simulink model "Progetto_predistorter_2020b"  (R2024b)
settings: Solver=VariableStepAuto  StartTime=0.0  StopTime=30  RelTol=1e-3
libraries: commrflib2 x4, commfilt2 x1
settings Model: Creator=babu9  LastModifiedBy=giorgiomessina
settings SolverCC: AlgebraicLoopSolver=TrustRegion
settings RTWCC: GPUComputeCapability=3.5  DLArmComputeVersion=19.05

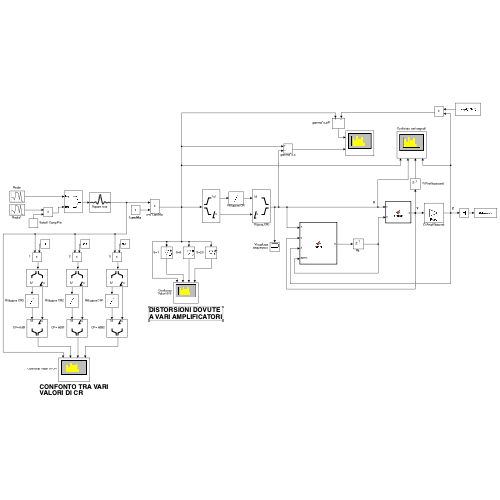
[thumbnail: Simulink's stored preview of the top-level diagram]
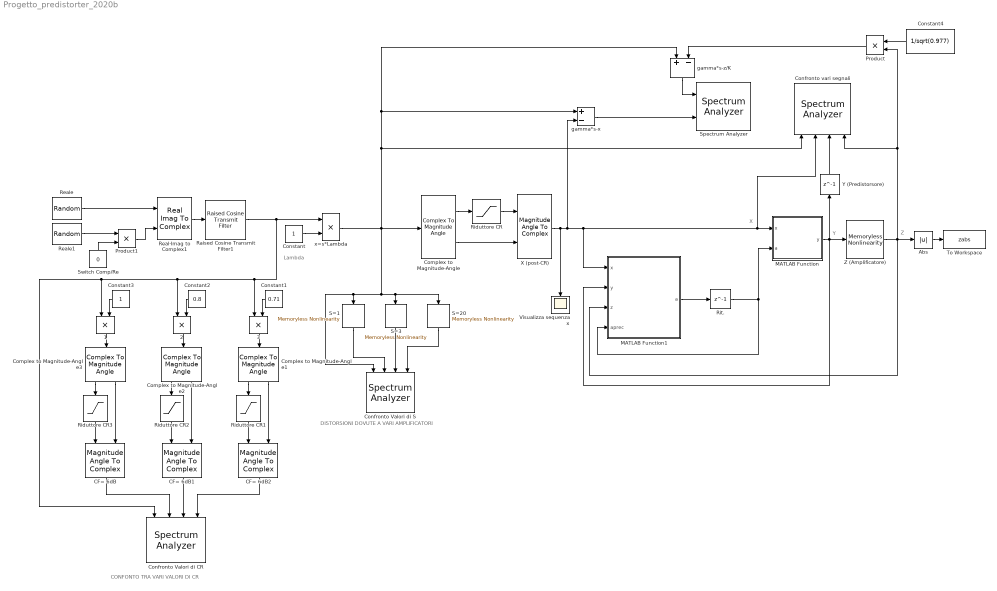
== system Progetto_predistorter_2020b ==
  note: DISTORSIONI DOVUTE
      | A VARI AMPLIFICATORI
  note: X
  note: Z
  note: Y
  note: Lambda
  note: CONFONTO TRA VARI
      | VALORI DI CR
  " X (post-CR)" : MagnitudeAngleToComplex
  1 : Product
  2 : Product
  3 : Product
  Abs : Abs  SaturateOnIntegerOverflow=off
  CF= 6dB : MagnitudeAngleToComplex
  CF= 6dB1 : MagnitudeAngleToComplex
  CF= 6dB2 : MagnitudeAngleToComplex
  Complex to Magnitude-Angle{,1..3} (4 alike) : ComplexToMagnitudeAngle
  Confronto Valori di S : SpectrumAnalyzer  NumInputPorts=4  WindowPosition=[320.000000,200.000000,800.000000,500.000000,]  ScopeFrameLocation=window  AveragingMethod=Exponential  YLimits=[-123.86285109,20.50800474]  ShowLegend=on  ChannelNames="[\"\"]"  AllowFFTLengthLessThanSamplesPerUpdate=on  DefaultConfigurationName=spbscopes.SpectrumAnalyzerBlockCfg
      settings: OpenAtSimulationStart=off
  Confronto Valori di CR : SpectrumAnalyzer  NumInputPorts=4  WindowPosition=[320.000000,200.000000,800.000000,500.000000,]  ScopeFrameLocation=window  AveragingMethod=Exponential  YLimits=[-123.86285109,20.50800474]  ShowLegend=on  ChannelNames="[\"\"]"  AllowFFTLengthLessThanSamplesPerUpdate=on  DefaultConfigurationName=spbscopes.SpectrumAnalyzerBlockCfg
      settings: OpenAtSimulationStart=off
  Confronto vari segnali : SpectrumAnalyzer  NumInputPorts=4  WindowPosition=[320.000000,200.000000,800.000000,500.000000,]  ScopeFrameLocation=window  AveragingMethod=Exponential  YLimits=[-128.13154737,58.92627127]  ShowLegend=on  ChannelNames="[\"\"]"  AllowFFTLengthLessThanSamplesPerUpdate=on  DefaultConfigurationName=spbscopes.SpectrumAnalyzerBlockCfg
      settings: OpenAtSimulationStart=off
  Constant : Constant
  Constant1 : Constant  Value=0.71
  Constant2 : Constant  Value=0.8
  Constant3 : Constant
  Constant4 : Constant  Value=1/sqrt(0.977)
  MATLAB Function : MATLAB Function  TreatAsAtomicUnit=on
  MATLAB Function1 : MATLAB Function  TreatAsAtomicUnit=on
  Product : Product
  Product1 : Product
  Raised Cosine Transmit Filter1 : commfilt2/Raised Cosine Transmit Filter  filtType=Square root  R=0.25  filtSpan=100  N=8  filterGain=1  RateOptions=Allow multirate processing  framing=Mute  checkCoeff=off  variableName=TransmitFilter1  checkGain=Normalized  sampMode=Mute  saveAsFlag=0  currentFiltSpan=10  D=(10)/2  launchFVT=on  roundingMode=Floor  overflowMode=off  coeffDataTypeStr=Inherit: Same word length as input  coeffMin=[]  coeffMax=[]  coeffLastDataTypeStr=Inherit: Same word length as input  outputDataTypeStr=Inherit: Same as accumulator  outputMin=[]  outputMax=[]  outputLastDataTypeStr=Inherit: Same as accumulator
  Real-Imag to Complex1 : RealImagToComplex
  Reale : RandomNumber  Variance=2  Seed=3742346792324  SampleTime=0.001
  Reale1 : RandomNumber  Seed=4387648932479  SampleTime=0.001
  Riduttore CR{,1..3} (4 alike) : Saturate  UpperLimit=1  LowerLimit=-1
  Rit. : Delay  DelayLength=1  InitialCondition=ones(51,1)
  S=1 : commrflib2/Memoryless Nonlinearity  Model=modified-rapp  Gain=0  Nonlinearity=IIP3  IIP3=Inf  OIP3=Inf  IP1dB=Inf  OP1dB=Inf  IPsat=Inf  OPsat=Inf  Table=[ -25, 5, -1; -10, 20, -2; 0, 27, 5; 5, 28, 12 ]  MagnitudeGainDB=0  Vsat=1  MagnitudeSmooth=1  PhaseGainRadian=0  PhaseSaturation=1  PhaseSmooth=3.43  InputScaleDB=0  AmAmParameters=[ 2.1587, 1.1517 ]  AmPmParameters=[ 4.0033, 9.1040 ]  OutputScaleDB=0  ReferenceLoad=1  SimulateUsing=Code generation
  S=20 : commrflib2/Memoryless Nonlinearity  Model=modified-rapp  Gain=0  Nonlinearity=IIP3  IIP3=Inf  OIP3=Inf  IP1dB=Inf  OP1dB=Inf  IPsat=Inf  OPsat=Inf  Table=[ -25, 5, -1; -10, 20, -2; 0, 27, 5; 5, 28, 12 ]  MagnitudeGainDB=0  Vsat=1  MagnitudeSmooth=20  PhaseGainRadian=0  PhaseSaturation=1  PhaseSmooth=3.43  InputScaleDB=0  AmAmParameters=[ 2.1587, 1.1517 ]  AmPmParameters=[ 4.0033, 9.1040 ]  OutputScaleDB=0  ReferenceLoad=1  SimulateUsing=Code generation
  S=3 : commrflib2/Memoryless Nonlinearity  Model=modified-rapp  Gain=0  Nonlinearity=IIP3  IIP3=Inf  OIP3=Inf  IP1dB=Inf  OP1dB=Inf  IPsat=Inf  OPsat=Inf  Table=[ -25, 5, -1; -10, 20, -2; 0, 27, 5; 5, 28, 12 ]  MagnitudeGainDB=0  Vsat=1  MagnitudeSmooth=3  PhaseGainRadian=0  PhaseSaturation=1  PhaseSmooth=3.43  InputScaleDB=0  AmAmParameters=[ 2.1587, 1.1517 ]  AmPmParameters=[ 4.0033, 9.1040 ]  OutputScaleDB=0  ReferenceLoad=1  SimulateUsing=Code generation
  Spectrum Analyzer : SpectrumAnalyzer  NumInputPorts=2  WindowPosition=[321.000000,207.000000,800.000000,500.000000,]  ScopeFrameLocation=window  AveragingMethod=Exponential  YLimits=[-53.51673738,7.37726191]  ShowLegend=on  ChannelNames="[\"\"]"  AllowFFTLengthLessThanSamplesPerUpdate=on  DefaultConfigurationName=spbscopes.SpectrumAnalyzerBlockCfg
      settings: OpenAtSimulationStart=off
  Switch Comp/Re : Constant  Value=0
  To Workspace : ToWorkspace  VariableName=zabs  SampleTime=-1
      settings: Save2DSignal=2-D array (concatenate along first dimension)
  Visualizza sequenza x : Scope
  Y (Predistorsore) : Delay  DelayLength=1  InitialCondition=0
  Z (Amplificatore) : commrflib2/Memoryless Nonlinearity  Model=modified-rapp  Gain=0  Nonlinearity=IIP3  IIP3=Inf  OIP3=Inf  IP1dB=Inf  OP1dB=Inf  IPsat=Inf  OPsat=Inf  Table=[ -25, 5, -1; -10, 20, -2; 0, 27, 5; 5, 28, 12 ]  MagnitudeGainDB=0  Vsat=1  MagnitudeSmooth=3  PhaseGainRadian=0  PhaseSaturation=1  PhaseSmooth=3.43  InputScaleDB=0  AmAmParameters=[ 2.1587, 1.1517 ]  AmPmParameters=[ 4.0033, 9.1040 ]  OutputScaleDB=0  ReferenceLoad=1  SimulateUsing=Code generation
  gamma*s-x : Sum  Inputs=+-
  gamma*s-z/K : Sum  Inputs=+-
  x=s*Lambda : Product
  wires:
  Reale/1 -> Real-Imag to Complex1/1
  Constant/1 -> x=s*Lambda/2
  Riduttore CR/1 -> " X (post-CR)"/1
  Complex to Magnitude-Angle/1 -> Riduttore CR/1
  Complex to Magnitude-Angle/2 -> " X (post-CR)"/2
  Z (Amplificatore)/1 -> MATLAB Function1/3(z), Abs/1, Confronto vari segnali/4, Product/2
  MATLAB Function1/1(a) -> Rit./1
  Rit./1 -> MATLAB Function/2(a), MATLAB Function1/4(aprec)
  Reale1/1 -> Product1/1
  Switch Comp/Re/1 -> Product1/2
  Product1/1 -> Real-Imag to Complex1/2
  S=1/1 -> Confronto Valori di S/2
  S=3/1 -> Confronto Valori di S/3
  S=20/1 -> Confronto Valori di S/4
  Abs/1 -> To Workspace/1
  MATLAB Function/1(y) -> Y (Predistorsore)/1, Z (Amplificatore)/1, MATLAB Function1/2(y)
  Y (Predistorsore)/1 -> Confronto vari segnali/3
  x=s*Lambda/1 -> gamma*s-x/1, gamma*s-z/K/1, Confronto vari segnali/1, Complex to Magnitude-Angle/1, Confronto Valori di S/1, S=1/1, S=20/1, S=3/1
  Constant4/1 -> Product/1
  Product/1 -> gamma*s-z/K/2
  gamma*s-z/K/1 -> Spectrum Analyzer/1
  gamma*s-x/1 -> Spectrum Analyzer/2
  Complex to Magnitude-Angle1/2 -> CF= 6dB2/2
  CF= 6dB1/1 -> Confronto Valori di CR/3
  Complex to Magnitude-Angle2/2 -> CF= 6dB1/2
  3/1 -> Complex to Magnitude-Angle1/1
  CF= 6dB2/1 -> Confronto Valori di CR/4
  CF= 6dB/1 -> Confronto Valori di CR/2
  Riduttore CR1/1 -> CF= 6dB2/1
  Complex to Magnitude-Angle3/2 -> CF= 6dB/2
  Riduttore CR2/1 -> CF= 6dB1/1
  Complex to Magnitude-Angle3/1 -> Riduttore CR3/1
  Complex to Magnitude-Angle1/1 -> Riduttore CR1/1
  Complex to Magnitude-Angle2/1 -> Riduttore CR2/1
  Constant1/1 -> 3/2
  1/1 -> Complex to Magnitude-Angle3/1
  2/1 -> Complex to Magnitude-Angle2/1
  Riduttore CR3/1 -> CF= 6dB/1
  Constant3/1 -> 1/2
  Constant2/1 -> 2/2
  Raised Cosine Transmit Filter1/1 -> x=s*Lambda/1, 2/1, 1/1, Confronto Valori di CR/1, 3/1
  Real-Imag to Complex1/1 -> Raised Cosine Transmit Filter1/1
  " X (post-CR)"/1 -> Visualizza sequenza x/1, MATLAB Function/1(x), Confronto vari segnali/2, MATLAB Function1/1(x), gamma*s-x/2

== matlab function Progetto_predistorter_2020b/MATLAB Function1 ==
  data: x input; a output; y input; z input; aprec input
function a=adapt(x,y,z,aprec)
   
    N=16; % detto dal prof: utilizzare pochi intervalli (es. 16 per ottenere 32)
    gamma=0.4;
    xmax=1;
    K=sqrt(0.977);
    delta=abs(xmax)/(2*N) ; % interval's size
    
    if(abs(x) > xmax)
        n=N;
    else
        n  = (abs(x)- (mod(abs(x),delta)) ) / delta; %vettore degli indici di aprec
    end
    
    aprec(n+1)=real(   aprec(n+1)-gamma*(z-K*x)*conj(x*z/y)   );
    a=aprec;

end

% La formula di "n" per abs(x)<=xmax serve ad identificare l'indice (del
% vettore "a" di valori da introdurre nel predistorsore) in cui si colloca
% il valore abs(x), data la sequenza in ingresso x.

% mod(abs(x),delta)
% serve a calcolare il discostamento tra abs(x) e
% l'intervallo più vicino ad esso.

% abs(x) - (mod(abs(x),delta)
% fornisce il primo valore dell'intervallo a cui appartiene abs(x).

% (abs(x) - (mod(abs(x),delta)) / delta
% ricava semplicemente il numero di intervalli da "saltare" (a partire da 0)
% per raggiungere quello identificato precedentemente.

== matlab function Progetto_predistorter_2020b/MATLAB Function ==
  data: x input; y output; a input

function y=predist(x,a)

    N=16;
    xmax=1;
    delta = abs(xmax)/(2*N); % interval's size 

    if(abs(x) >= xmax)
        P=a(N+1);
    else
        n = floor(((abs(x)-(mod(abs(x),delta)))/delta)/2) ;
        P = (abs(x) - (2*n+1)*delta)*(a(n+2)-a(n+1))/(2*delta) + (a(n+2)+a(n+1))/2 ;
    end
    
    y = P*x;
end
